simulink model "KStestsimulate"  (Simulink 7.8)
settings: Solver=ode45  StartTime=0.0  StopTime=10.0  RelTol=1e-3
values from neighbouring files (symbols this model uses):
  Dtab = 0.565    [KS_data.mat]
  R = [0.12 0.87 0.85 0.05 0.21]    [KS_data.mat]
libraries: simulink x1
settings Model: Creator=Windows  LastModifiedBy=Windows

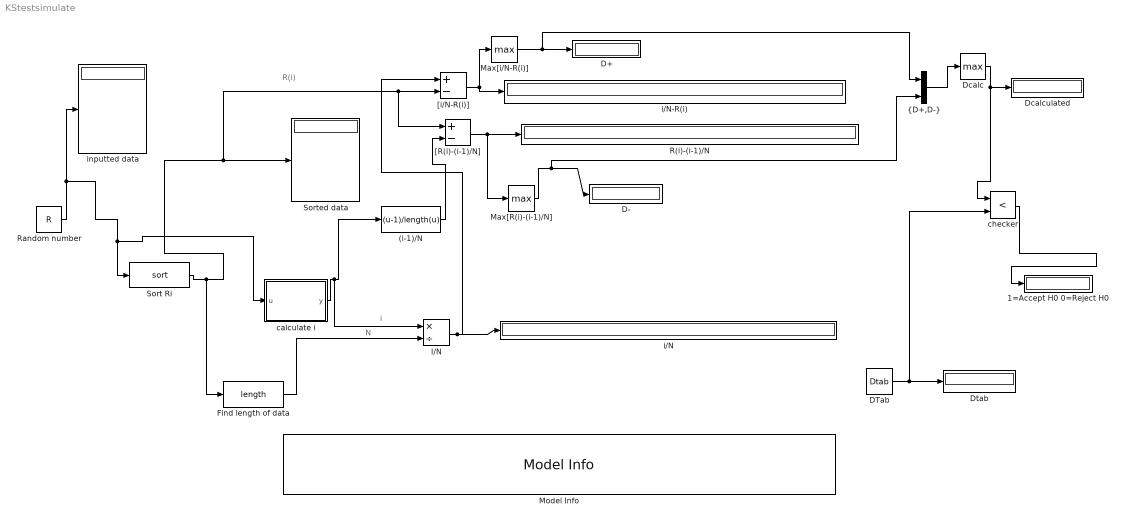
== system KStestsimulate ==
  note: i
  note: N
  note: R(i)
  (i-1)/N : MATLABFcn  MATLABFcn=(u-1)/length(u)
  1=Accept H0 0=Reject H0 : Display
  D+ : Display
  D- : Display
  DTab : Constant  Value=Dtab
  Dcalc : MinMax  Function=max
  Dcalculated : Display
  Dtab : Display
  Find length of data : MATLABFcn  MATLABFcn=length
  I/N : Product  Inputs=*/
  Max[R(i)-(i-1)/N] : MinMax  Function=max
  Max[i/N-R(i)] : MinMax  Function=max
  Model Info : simulink/Model-Wide Utilities/Model Info  InitialBlockCM=None  BlockCM=None  Frame=on  DisplayStringWithTags=|  HorizontalTextAlignment=Center  LeftAlignmentValue=0.5  SourceBlockDiagram=KStestsimulate  TagMaxNumber=20
      | Model Info
      | %<ModelName>
      | %<Created>
      | KS test is the test to determine whether the inputted random number are uniformly distributed or not.
  R(i)-(i-1)/N : Display
  Random number : Constant  Value=R
  Sort Ri : MATLABFcn  MATLABFcn=sort
  Sorted data : Display
  "[R(i)-(i-1)/N]" : Sum  Inputs=+-
  "[i/N-R(i)]" : Sum  Inputs=+-
  calculate i : MATLAB Function  TreatAsAtomicUnit=on
  checker : RelationalOperator  Operator=<  OutDataTypeStr=boolean
  i/N : Display
  i/N-R(i) : Display
  inputted data : Display
  "{D+,D-}" : Concatenate  Mode=Vector
  wires:
  Random number/1 -> inputted data/1, Sort Ri/1, calculate i/1(u)
  Sort Ri/1 -> Find length of data/1, Sorted data/1, "[i/N-R(i)]"/2, "[R(i)-(i-1)/N]"/1
  Find length of data/1 -> I/N/2
  calculate i/1(y) -> I/N/1, (i-1)/N/1
  I/N/1 -> "[i/N-R(i)]"/1, i/N/1
  "[i/N-R(i)]"/1 -> i/N-R(i)/1, Max[i/N-R(i)]/1
  "[R(i)-(i-1)/N]"/1 -> R(i)-(i-1)/N/1, Max[R(i)-(i-1)/N]/1
  Max[R(i)-(i-1)/N]/1 -> D-/1, "{D+,D-}"/2
  Max[i/N-R(i)]/1 -> D+/1, "{D+,D-}"/1
  "{D+,D-}"/1 -> Dcalc/1
  checker/1 -> 1=Accept H0 0=Reject H0/1
  DTab/1 -> Dtab/1, checker/2
  Dcalc/1 -> checker/1, Dcalculated/1
  (i-1)/N/1 -> "[R(i)-(i-1)/N]"/2

== matlab function calculate i ==
  data: u input double; y output double
function y = fcn(u)
%#codegen

 y = zeros(1,length(u));
for k=1:1:length(u)
    y(k)=k;
end
